simulink model "test_3ph_3w_transformer"  (R2018b)
settings: Solver=FixedStepDiscrete  StartTime=0.0  StopTime=1  RelTol=1e-3
undefined symbols (not defined in the file): S2
libraries: powerlib x11, typhoonHILlib x6
settings Model: Creator=USER  LastModifiedBy=USER

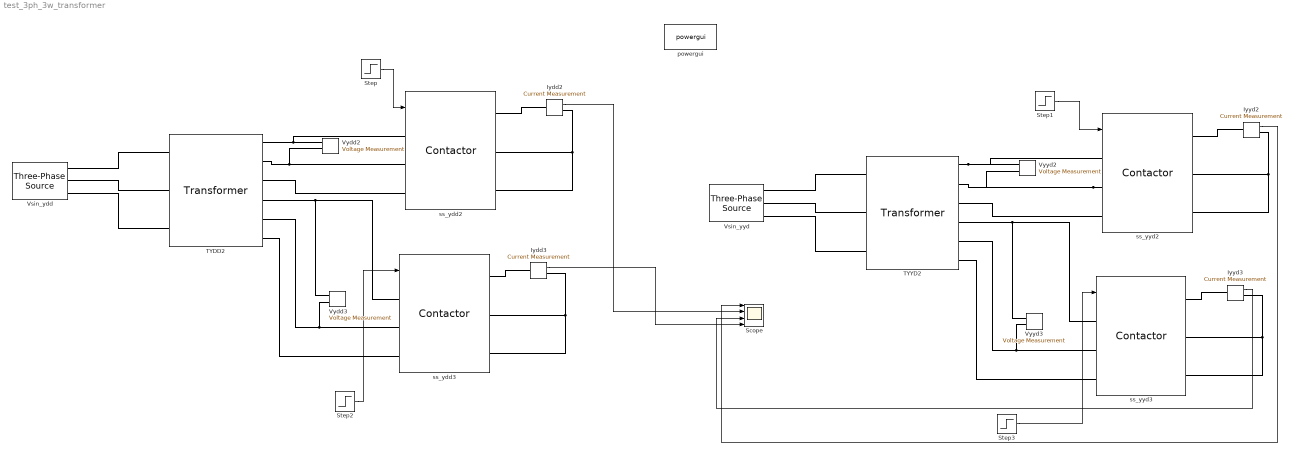
== system test_3ph_3w_transformer ==
  Iydd2 : powerlib/Measurements/Current Measurement  PhasorSimulation=off  OutputType=Complex  PSBequivalent=0
  Iydd3 : powerlib/Measurements/Current Measurement  PhasorSimulation=off  OutputType=Complex  PSBequivalent=0
  Iyyd2 : powerlib/Measurements/Current Measurement  PhasorSimulation=off  OutputType=Complex  PSBequivalent=0
  Iyyd3 : powerlib/Measurements/Current Measurement  PhasorSimulation=off  OutputType=Complex  PSBequivalent=0
  Scope : Scope  NumInputPorts=4
  Step{,1..3} (4 alike) : Step  Time=0.01  SampleTime=0
  TYDD2 : typhoonHILlib/Transformer  TransfType=Three-Phase Three Windings  Sn=160000.0  fn=50  Rm=10e3  Lm=300.0  sat_toggle=off  flux_vec=[0, 0.001, 0.005]  i_vec=[0, 1, 2]  n1=1  n2=1  coup12=off  coup13=off  coup14=off  units=SI  conn_1=Wye  V1=400  R1=4  L1=0.01  I1=0  conn_2=Delta  V2=173.20  R2=1.6875  L2=0.01125  I2=0  conn_3=Delta  V3=115.47  R3=0.5  L3=0.0075  I3=0  conn_4=Wye  V4=100  R4=0.1  L4=1e-3  I4=0  toggle_init=on  old_pat=typhoonPatterns/TP 3W Transformer  old_size=145,176  model_loaded=off
      settings: SourceProductName=Typhoon HIL
  TYYD2 : typhoonHILlib/Transformer  TransfType=Three-Phase Three Windings  Sn=160000.0  fn=50  Rm=10e3  Lm=300  sat_toggle=off  flux_vec=[0, 0.001, 0.005]  i_vec=[0, 1, 2]  n1=1  n2=1  coup12=off  coup13=off  coup14=off  units=SI  conn_1=Wye  V1=400  R1=4  L1=1e-2  I1=0  conn_2=Wye  V2=300  R2=1.6875  L2=0.01125  I2=0  conn_3=Delta  V3=115.47  R3=0.5  L3=0.0075  I3=0  conn_4=Wye  V4=100  R4=0.1  L4=1e-3  I4=0  toggle_init=on  old_pat=typhoonPatterns/TP 3W Transformer  old_size=145,176  model_loaded=off
      settings: SourceProductName=Typhoon HIL
  Vsin_ydd : powerlib/Electrical Sources/Three-Phase Source  InternalConnection=Yg  VoltagePhases=off  Voltage=1000  PhaseAngle=0  Voltage_phases=[25e3 25e3 25e3]/sqrt(3)  PhaseAngles_phases=[0 -120 +120]  Frequency=50  NonIdealSource=on  SpecifyImpedance=off  Resistance=0  Inductance=0  ShortCircuitLevel=100e6  BaseVoltage=0  XRratio=7  BusType=swing  Pref=10e3  Qref=0  Prefabc=[10e3, 10e3, 10e3]  Qrefabc=[0, 0, 0]  Qmin=-inf  Qmax=inf
  Vsin_yyd : powerlib/Electrical Sources/Three-Phase Source  InternalConnection=Yg  VoltagePhases=off  Voltage=1000  PhaseAngle=0  Voltage_phases=[25e3 25e3 25e3]/sqrt(3)  PhaseAngles_phases=[0 -120 +120]  Frequency=50  NonIdealSource=on  SpecifyImpedance=off  Resistance=0  Inductance=0  ShortCircuitLevel=100e6  BaseVoltage=0  XRratio=7  BusType=swing  Pref=10e3  Qref=0  Prefabc=[10e3, 10e3, 10e3]  Qrefabc=[0, 0, 0]  Qmin=-inf  Qmax=inf
  Vydd2 : powerlib/Measurements/Voltage Measurement  PhasorSimulation=off  OutputType=Complex  PSBequivalent=0
  Vydd3 : powerlib/Measurements/Voltage Measurement  PhasorSimulation=off  OutputType=Complex  PSBequivalent=0
  Vyyd2 : powerlib/Measurements/Voltage Measurement  PhasorSimulation=off  OutputType=Complex  PSBequivalent=0
  Vyyd3 : powerlib/Measurements/Voltage Measurement  PhasorSimulation=off  OutputType=Complex  PSBequivalent=0
  powergui : powerlib/powergui  Priority=1  SimulationMode=Discrete  SampleTime=1e-6  frequency=60  Iterations=50  frequencyindice=50  Pbase=100e6  ErrMax=1e-4  UnitsV=kV  UnitsW=MW  buscounter=0  FunctionMessages=off  echomessages=off  EnableUseOfTLC=off  CurrentSourceSwitches=off  DisableSnubberDevices=off  DisableRonSwitches=off  DisableVfSwitches=off  DisplayEquations=off  SolverType=Tustin/Backward Euler (TBE)  Interpol=off  ExternalGateDelay=off  methode=off  Ts=100  x0status=blocks  SPID=on  SwTol=0  HookPort=off  RestoreLinks=warning  ResistiveCurrentMeasurement=off  Frange=[0:2:500]  Ylog=off  Xlog=on  ShowGrid=off  save=off  variable=ZData  structure=0  ZoomFFT=off  StartTime=0.0  cycles=1  DisplayStyle=1  fundamental=60  FreqAxis=off  MaxFrequency=1000  frequencyindicesteady=1  RmsSteady=1  display=off
  ss_ydd2 : typhoonHILlib/Contactor  ContType=Triple Pole Single Throw  init_state=Off / S2  s1_logic=Active-high  di_1=1  tr1_delay=0  tr2_delay=0  r_on=0.001  v_f=0  r_s=1e4  c_s=inf  s0=0  toggle_init=on  old_pat=typhoonPatterns/TPST Contactor  old_size=140,185  model_loaded=off
      settings: SourceProductName=Typhoon HIL
  ss_ydd3 : typhoonHILlib/Contactor  ContType=Triple Pole Single Throw  init_state=Off / S2  s1_logic=Active-high  di_1=1  tr1_delay=0  tr2_delay=0  r_on=0.001  v_f=0  r_s=1e4  c_s=inf  s0=0  toggle_init=on  old_pat=typhoonPatterns/TPST Contactor  old_size=140,185  model_loaded=off
      settings: SourceProductName=Typhoon HIL
  ss_yyd2 : typhoonHILlib/Contactor  ContType=Triple Pole Single Throw  init_state=Off / S2  s1_logic=Active-high  di_1=1  tr1_delay=0  tr2_delay=0  r_on=0.001  v_f=0  r_s=1e4  c_s=inf  s0=0  toggle_init=on  old_pat=typhoonPatterns/TPST Contactor  old_size=140,185  model_loaded=off
      settings: SourceProductName=Typhoon HIL
  ss_yyd3 : typhoonHILlib/Contactor  ContType=Triple Pole Single Throw  init_state=Off / S2  s1_logic=Active-high  di_1=1  tr1_delay=0  tr2_delay=0  r_on=0.001  v_f=0  r_s=1e4  c_s=inf  s0=0  toggle_init=on  old_pat=typhoonPatterns/TPST Contactor  old_size=140,185  model_loaded=off
      settings: SourceProductName=Typhoon HIL
  wires:
  Step/1 -> ss_ydd2/1
  Step1/1 -> ss_yyd2/1
  Step2/1 -> ss_ydd3/1
  Step3/1 -> ss_yyd3/1
  Iydd3/1 -> Scope/4
  Iydd2/1 -> Scope/2
  Iyyd2/1 -> Scope/1
  Iyyd3/1 -> Scope/3
  connections:
  Vsin_ydd/RConn1 -- TYDD2/LConn1
  Vsin_ydd/RConn2 -- TYDD2/LConn2
  TYDD2/RConn2 -- Vydd2/LConn2 -- ss_ydd2/LConn2
  ss_ydd2/LConn1 -- Vydd2/LConn1 -- TYDD2/RConn1
  ss_ydd2/RConn1 -- Iydd2/LConn1
  Iydd2/RConn1 -- ss_ydd2/RConn2 -- ss_ydd2/RConn3
  Iydd3/RConn1 -- ss_ydd3/RConn2 -- ss_ydd3/RConn3
  ss_ydd3/RConn1 -- Iydd3/LConn1
  Vsin_ydd/RConn3 -- TYDD2/LConn3
  ss_ydd2/LConn3 -- TYDD2/RConn3
  TYDD2/RConn4 -- Vydd3/LConn1 -- ss_ydd3/LConn1
  TYDD2/RConn5 -- Vydd3/LConn2 -- ss_ydd3/LConn2
  TYDD2/RConn6 -- ss_ydd3/LConn3
  TYYD2/RConn4 -- Vyyd3/LConn1 -- ss_yyd3/LConn1
  TYYD2/RConn5 -- Vyyd3/LConn2 -- ss_yyd3/LConn2
  ss_yyd2/LConn2 -- Vyyd2/LConn2 -- TYYD2/RConn2
  Iyyd3/RConn1 -- ss_yyd3/RConn2 -- ss_yyd3/RConn3
  Iyyd2/RConn1 -- ss_yyd2/RConn2 -- ss_yyd2/RConn3
  TYYD2/RConn1 -- ss_yyd2/LConn1 -- Vyyd2/LConn1
  TYYD2/RConn6 -- ss_yyd3/LConn3
  ss_yyd2/RConn1 -- Iyyd2/LConn1
  ss_yyd2/LConn3 -- TYYD2/RConn3
  Vsin_yyd/RConn3 -- TYYD2/LConn3
  ss_yyd3/RConn1 -- Iyyd3/LConn1
  Vsin_yyd/RConn2 -- TYYD2/LConn2
  Vsin_yyd/RConn1 -- TYYD2/LConn1
